simulink model "test_vacc_pkt_10_1"  (Simulink 7.2)
settings: Solver=ode45  StartTime=0.0  StopTime=90000  RelTol=1e-3
libraries: xbsIndex_r4 x802, xps_library x17, casper_library_misc x10, xbsReplacements_r4 x9
(part 2 of 6)

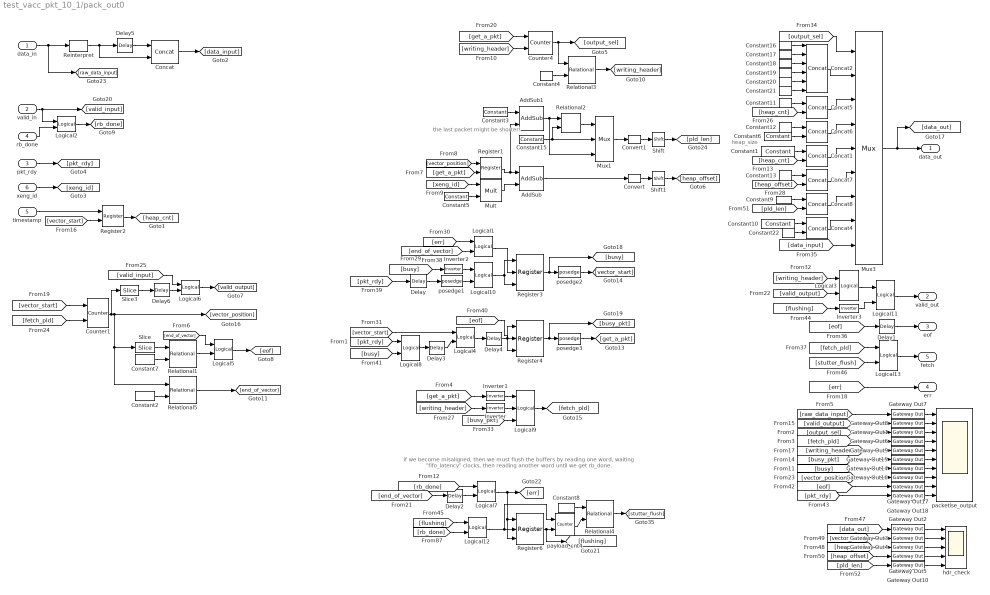
== system test_vacc_pkt_10_1/pack_out0 ==
  note: heap_size
  note: if we become misaligned,
      | then we must flush the buffers
      | by reading one word, waiting "fifo_latency" clocks,
      | then reading another word until we get rb_done.
  note: the last packet
      | might be shorter!
  data_in : Inport  OutDataType=sfix(16)  OutScaling=2^0
  valid_in : Inport  Port=2  OutDataType=sfix(16)  OutScaling=2^0
  pkt_rdy : Inport  Port=3  OutDataType=sfix(16)  OutScaling=2^0
  rb_done : Inport  Port=4  OutDataType=sfix(16)  OutScaling=2^0
  timestamp : Inport  Port=5  OutDataType=sfix(16)  OutScaling=2^0
  xeng_id : Inport  Port=6  OutDataType=sfix(16)  OutScaling=2^0
  AddSub : xbsIndex_r4/AddSub  mode=Addition  use_carryin=off  use_carryout=off  en=off  latency=1  precision=Full  arith_type=Unsigned  n_bits=16  bin_pt=14  quantization=Truncate  overflow=Wrap  dbl_ovrd=off  use_behavioral_HDL=on  hw_selection=Fabric  pipelined=off  block_type=addsub
  AddSub1 : xbsIndex_r4/AddSub  mode=Subtraction  use_carryin=off  use_carryout=off  en=off  latency=1  precision=Full  arith_type=Unsigned  n_bits=pkt_bits+4  bin_pt=0  quantization=Truncate  overflow=Wrap  dbl_ovrd=off  use_behavioral_HDL=on  hw_selection=Fabric  pipelined=off  block_type=addsub
  Concat{,1,4..8} (7 alike) : xbsIndex_r4/Concat  num_inputs=2  dbl_ovrd=off  block_type=concat
      settings: block_version=10.1.3
  Concat2 : xbsIndex_r4/Concat  num_inputs=6  dbl_ovrd=off  block_type=concat
      settings: block_version=10.1.3
  Constant1 : xbsIndex_r4/Constant  arith_type=Unsigned  const=5632 + 2^(spead_msw-spead_lsw-1)  n_bits=spead_msw-spead_lsw  bin_pt=0  explicit_period=on  period=1  equ=P=C  opselect=C  inp2=PCIN>>17  opr=+  inp1=P  carry=CIN  dbl_ovrd=off  block_type=constant
  Constant10 : xbsIndex_r4/Constant  arith_type=Unsigned  const=spead_item  n_bits=spead_msw-spead_lsw  bin_pt=0  explicit_period=on  period=1  equ=P=C  opselect=C  inp2=PCIN>>17  opr=+  inp1=P  carry=CIN  dbl_ovrd=off  block_type=constant
  Constant11 : xbsIndex_r4/Constant  arith_type=Unsigned  const=1 + 2^(spead_msw-spead_lsw-1)  n_bits=spead_msw-spead_lsw  bin_pt=0  explicit_period=on  period=1  equ=P=C  opselect=C  inp2=PCIN>>17  opr=+  inp1=P  carry=CIN  dbl_ovrd=off  block_type=constant
  Constant12 : xbsIndex_r4/Constant  arith_type=Unsigned  const="2 +  + 2^(spead_msw-spead_lsw-1)"  n_bits=spead_msw-spead_lsw  bin_pt=0  explicit_period=on  period=1  equ=P=C  opselect=C  inp2=PCIN>>17  opr=+  inp1=P  carry=CIN  dbl_ovrd=off  block_type=constant
  Constant13 : xbsIndex_r4/Constant  arith_type=Unsigned  const=3 + 2^(spead_msw-spead_lsw-1)  n_bits=spead_msw-spead_lsw  bin_pt=0  explicit_period=on  period=1  equ=P=C  opselect=C  inp2=PCIN>>17  opr=+  inp1=P  carry=CIN  dbl_ovrd=off  block_type=constant
  Constant15 : xbsIndex_r4/Constant  arith_type=Unsigned  const=(pkt_len*2)  n_bits=pkt_bits+2  bin_pt=0  explicit_period=on  period=1  equ=P=C  opselect=C  inp2=PCIN>>17  opr=+  inp1=P  carry=CIN  dbl_ovrd=off  block_type=constant
  Constant16 : xbsIndex_r4/Constant  arith_type=Unsigned  const=83  n_bits=8  bin_pt=0  explicit_period=on  period=1  equ=P=C  opselect=C  inp2=PCIN>>17  opr=+  inp1=P  carry=CIN  dbl_ovrd=off  block_type=constant
  Constant17 : xbsIndex_r4/Constant  arith_type=Unsigned  const=4  n_bits=8  bin_pt=0  explicit_period=on  period=1  equ=P=C  opselect=C  inp2=PCIN>>17  opr=+  inp1=P  carry=CIN  dbl_ovrd=off  block_type=constant
  Constant18 : xbsIndex_r4/Constant  arith_type=Unsigned  const=(spead_msw-spead_lsw)/8  n_bits=8  bin_pt=0  explicit_period=on  period=1  equ=P=C  opselect=C  inp2=PCIN>>17  opr=+  inp1=P  carry=CIN  dbl_ovrd=off  block_type=constant
  Constant19 : xbsIndex_r4/Constant  arith_type=Unsigned  const=spead_lsw/8  n_bits=8  bin_pt=0  explicit_period=on  period=1  equ=P=C  opselect=C  inp2=PCIN>>17  opr=+  inp1=P  carry=CIN  dbl_ovrd=off  block_type=constant
  Constant2 : xbsIndex_r4/Constant  arith_type=Unsigned  const=(vector_len)-1  n_bits=vector_bits+1  bin_pt=0  explicit_period=on  period=1  equ=P=C  opselect=C  inp2=PCIN>>17  opr=+  inp1=P  carry=CIN  dbl_ovrd=off  block_type=constant
  Constant20 : xbsIndex_r4/Constant  arith_type=Unsigned  const=0  n_bits=16  bin_pt=0  explicit_period=on  period=1  equ=P=C  opselect=C  inp2=PCIN>>17  opr=+  inp1=P  carry=CIN  dbl_ovrd=off  block_type=constant
  Constant21 : xbsIndex_r4/Constant  arith_type=Unsigned  const=6  n_bits=16  bin_pt=0  explicit_period=on  period=1  equ=P=C  opselect=C  inp2=PCIN>>17  opr=+  inp1=P  carry=CIN  dbl_ovrd=off  block_type=constant
  Constant22 : xbsIndex_r4/Constant  arith_type=Unsigned  const=0  n_bits=spead_lsw  bin_pt=0  explicit_period=on  period=1  equ=P=C  opselect=C  inp2=PCIN>>17  opr=+  inp1=P  carry=CIN  dbl_ovrd=off  block_type=constant
  Constant3 : xbsIndex_r4/Constant  arith_type=Unsigned  const=vector_len  n_bits=vector_bits+1  bin_pt=0  explicit_period=on  period=1  equ=P=C  opselect=C  inp2=PCIN>>17  opr=+  inp1=P  carry=CIN  dbl_ovrd=off  block_type=constant
  Constant4 : xbsIndex_r4/Constant  arith_type=Unsigned  const=7  n_bits=3  bin_pt=0  explicit_period=on  period=1  equ=P=C  opselect=C  inp2=PCIN>>17  opr=+  inp1=P  carry=CIN  dbl_ovrd=off  block_type=constant
  Constant5 : xbsIndex_r4/Constant  arith_type=Unsigned  const=vector_len  n_bits=vector_bits+1  bin_pt=0  explicit_period=on  period=1  equ=P=C  opselect=C  inp2=PCIN>>17  opr=+  inp1=P  carry=CIN  dbl_ovrd=off  block_type=constant
  Constant6 : xbsIndex_r4/Constant  arith_type=Unsigned  const=heap_len  n_bits=spead_lsw  bin_pt=0  explicit_period=on  period=1  equ=P=C  opselect=C  inp2=PCIN>>17  opr=+  inp1=P  carry=CIN  dbl_ovrd=off  block_type=constant
  Constant7 : xbsIndex_r4/Constant  arith_type=Unsigned  const=(pkt_len*2)-1  n_bits=pkt_bits+1  bin_pt=0  explicit_period=on  period=1  equ=P=C  opselect=C  inp2=PCIN>>17  opr=+  inp1=P  carry=CIN  dbl_ovrd=off  block_type=constant
  Constant8 : xbsIndex_r4/Constant  arith_type=Unsigned  const=1  n_bits=ceil(log2(fifo_latency))+1  bin_pt=0  explicit_period=on  period=1  equ=P=C  opselect=C  inp2=PCIN>>17  opr=+  inp1=P  carry=CIN  dbl_ovrd=off  block_type=constant
  Constant9 : xbsIndex_r4/Constant  arith_type=Unsigned  const=4 + 2^(spead_msw-spead_lsw-1)  n_bits=spead_msw-spead_lsw  bin_pt=0  explicit_period=on  period=1  equ=P=C  opselect=C  inp2=PCIN>>17  opr=+  inp1=P  carry=CIN  dbl_ovrd=off  block_type=constant
  Convert : xbsIndex_r4/Convert  arith_type=Unsigned  n_bits=spead_lsw  bin_pt=0  quantization=Truncate  overflow=Wrap  latency=0  dbl_ovrd=off  pipeline=off  block_type=convert
      settings: block_version=11.4
  Convert1 : xbsIndex_r4/Convert  arith_type=Unsigned  n_bits=spead_lsw  bin_pt=0  quantization=Truncate  overflow=Wrap  latency=0  dbl_ovrd=off  pipeline=off  block_type=convert
      settings: block_version=11.4
  Counter1 : xbsIndex_r4/Counter  cnt_type=Free Running  cnt_to=1023  operation=Up  start_count=0  cnt_by_val=1  arith_type=Unsigned  n_bits=vector_bits+1  bin_pt=0  load_pin=off  rst=on  en=on  explicit_period=on  period=1  dbl_ovrd=off  use_behavioral_HDL=off  implementation=Fabric  use_rpm=on  block_type=counter
      settings: xl_area=[0, 0, 0, 0, 0, 0, 0]
  Counter4 : xbsIndex_r4/Counter  cnt_type=Free Running  cnt_to=1023  operation=Up  start_count=0  cnt_by_val=1  arith_type=Unsigned  n_bits=3  bin_pt=0  load_pin=off  rst=on  en=on  explicit_period=on  period=1  dbl_ovrd=off  use_behavioral_HDL=off  implementation=Fabric  use_rpm=on  block_type=counter
      settings: xl_area=[0, 0, 0, 0, 0, 0, 0]
  Delay : xbsIndex_r4/Delay  en=off  latency=1  dbl_ovrd=off  reg_retiming=on  block_type=delay
      settings: block_version=11.4
  Delay{1..2,4,6} (4 alike) : xbsIndex_r4/Delay  en=off  latency=fifo_latency  dbl_ovrd=off  reg_retiming=on  block_type=delay
      settings: block_version=11.4
  Delay3 : xbsIndex_r4/Delay  en=off  latency=1  dbl_ovrd=off  reg_retiming=on  block_type=delay
      settings: block_version=11.4
  Delay5 : xbsIndex_r4/Delay  en=off  latency=1  dbl_ovrd=off  reg_retiming=on  block_type=delay
      settings: block_version=11.4
  Gateway Out{1..10,14..18} (15 alike) : xbsIndex_r4/Gateway Out  hdl_port=on  timing_constraint=None  locs_specified=off  LOCs={}  block_type=gatewayout
      settings: infoedit="Gateway out block.  Converts Xilinx fixed point inputs into ouputs of type Simulink integer, double, or fixed point.<P><P>Hardware notes:  In hardware these blocks become top level output ports or are discarded, depending on how they are configured."  xl_area=[0, 0, 0, 0, 0, 0, 0]  block_version=10.1.3
  Inverter{,1..3} (4 alike) : xbsIndex_r4/Inverter  en=off  latency=0  dbl_ovrd=off  block_type=inv
      settings: block_version=11.4
  Logical{1,3..5,13} (5 alike) : xbsIndex_r4/Logical  logical_function=OR  inputs=2  en=off  latency=0  precision=Full  arith_type=Unsigned  n_bits=8  bin_pt=2  align_bp=on  dbl_ovrd=off  block_type=logical
      settings: xl_area=[0, 0, 0, 0, 0, 0, 0]
  Logical{2,6,8,10..12} (6 alike) : xbsIndex_r4/Logical  logical_function=AND  inputs=2  en=off  latency=0  precision=Full  arith_type=Unsigned  n_bits=8  bin_pt=2  align_bp=on  dbl_ovrd=off  block_type=logical
      settings: xl_area=[0, 0, 0, 0, 0, 0, 0]
  Logical7 : xbsIndex_r4/Logical  logical_function=XOR  inputs=2  en=off  latency=0  precision=Full  arith_type=Unsigned  n_bits=8  bin_pt=2  align_bp=on  dbl_ovrd=off  block_type=logical
      settings: xl_area=[0, 0, 0, 0, 0, 0, 0]
  Logical9 : xbsIndex_r4/Logical  logical_function=AND  inputs=3  en=off  latency=0  precision=Full  arith_type=Unsigned  n_bits=8  bin_pt=2  align_bp=on  dbl_ovrd=off  block_type=logical
      settings: xl_area=[0, 0, 0, 0, 0, 0, 0]
  Mult : xbsIndex_r4/Mult  precision=Full  arith_type="Signed  (2's comp)"  n_bits=16  bin_pt=14  quantization=Truncate  overflow=Wrap  en=off  latency=3  dbl_ovrd=off  use_behavioral_HDL=on  opt=Speed  use_embedded=on  optimum_pipeline=on  pipeline=on  use_rpm=on  placement_style=Triangular  block_type=mult
      settings: block_version=11.4
  Mux1 : xbsIndex_r4/Mux  inputs=2  en=off  latency=1  precision=Full  arith_type="Signed  (2's comp)"  n_bits=8  bin_pt=2  quantization=Truncate  overflow=Wrap  dbl_ovrd=off  block_type=mux
      settings: xl_area=[0, 0, 0, 0, 0, 0, 0]
  Mux3 : xbsIndex_r4/Mux  inputs=8  en=off  latency=0  precision=Full  arith_type="Signed  (2's comp)"  n_bits=8  bin_pt=2  quantization=Truncate  overflow=Wrap  dbl_ovrd=off  block_type=mux
      settings: xl_area=[0, 0, 0, 0, 0, 0, 0]
  Register1 : xbsIndex_r4/Register  init=0  rst=off  en=on  dbl_ovrd=off  block_type=register
  Register2 : xbsIndex_r4/Register  init=0  rst=off  en=on  dbl_ovrd=off  block_type=register
  Register3 : xbsIndex_r4/Register  init=0  rst=on  en=on  dbl_ovrd=off  block_type=register
  Register4 : xbsIndex_r4/Register  init=0  rst=on  en=on  dbl_ovrd=off  block_type=register
  Register6 : xbsIndex_r4/Register  init=0  rst=on  en=on  dbl_ovrd=off  block_type=register
      settings: xl_area=[0, 0, 0, 0, 0, 0, 0]
  Reinterpret : xbsIndex_r4/Reinterpret  force_arith_type=on  arith_type=Unsigned  force_bin_pt=on  bin_pt=0  block_type=reinterpret
      settings: infoedit="Changes signal type without altering the binary representation.   You can changed the signal between signed and unsigned, and relocate the binary point.<br><br>Hardware notes: In hardware this block costs nothing.<br><br>Example:  Suppose the input is 6 bits wide, signed, with 2 fractional bits, and the output is forced to unsigned with 0 fractional bits.  Then an input of -2.0 (1110.00 in binary 2's complement) becomes an output of 56 (111000 in binary)."
  Relational1 : xbsIndex_r4/Relational  mode=a=b  en=off  latency=0  dbl_ovrd=off  block_type=relational
      settings: xl_area=[0, 0, 0, 0, 0, 0, 0]  block_version=10.1.3
  Relational2 : xbsIndex_r4/Relational  mode=a<b  en=off  latency=0  dbl_ovrd=off  block_type=relational
      settings: xl_area=[0, 0, 0, 0, 0, 0, 0]  block_version=10.1.3
  Relational3 : xbsIndex_r4/Relational  mode=a<b  en=off  latency=0  dbl_ovrd=off  block_type=relational
      settings: xl_area=[0, 0, 0, 0, 0, 0, 0]  block_version=10.1.3
  Relational4 : xbsIndex_r4/Relational  mode=a=b  en=off  latency=0  dbl_ovrd=off  block_type=relational
      settings: xl_area=[0, 0, 0, 0, 0, 0, 0]  block_version=10.1.3
  Relational5 : xbsIndex_r4/Relational  mode=a=b  en=off  latency=0  dbl_ovrd=off  block_type=relational
      settings: xl_area=[0, 0, 0, 0, 0, 0, 0]  block_version=10.1.3
  Shift : xbsIndex_r4/Shift  shift_dir=Left  shift_bits=2  en=off  latency=0  precision=Full  arith_type="Signed  (2's comp)"  n_bits=16  bin_pt=14  quantization=Truncate  overflow=Wrap  dbl_ovrd=off  block_type=shift
  Shift1 : xbsIndex_r4/Shift  shift_dir=Left  shift_bits=2  en=off  latency=0  precision=Full  arith_type="Signed  (2's comp)"  n_bits=16  bin_pt=14  quantization=Truncate  overflow=Wrap  dbl_ovrd=off  block_type=shift
  Slice : xbsIndex_r4/Slice  nbits=pkt_bits+1  boolean_output=off  mode=Lower Bit Location + Width  bit1=0  base1=MSB of Input  bit0=0  base0=LSB of Input  dbl_ovrd=off  block_type=slice
  Slice3 : xbsIndex_r4/Slice  nbits=1  boolean_output=on  mode=Lower Bit Location + Width  bit1=0  base1=MSB of Input  bit0=0  base0=LSB of Input  dbl_ovrd=off  block_type=slice
  hdr_check : Scope  NumInputPorts=5
      settings: YMin=0~0~0~0~920  YMax=1e+19~1~17500~3250~1030  SaveName=ScopeData12
  packetise_output : Scope  NumInputPorts=10
      settings: YMin=1000~-1~7~-1~-1~-1~-1~1024~-1~-1  YMax=1000~1~7~1~1~1~1~1024~1~1
  payload_cnt4 : xbsIndex_r4/Counter  cnt_type=Count Limited  cnt_to=max((fifo_latency + 1),2)  operation=Up  start_count=0  cnt_by_val=1  arith_type=Unsigned  n_bits=ceil(log2(fifo_latency))+1  bin_pt=0  load_pin=off  rst=on  en=on  explicit_period=on  period=1  dbl_ovrd=off  use_behavioral_HDL=off  implementation=Fabric  use_rpm=on  block_type=counter
      settings: xl_area=[0, 0, 0, 0, 0, 0, 0]
  posedge1 : casper_library_misc/posedge  Tag=Rising Edge Detector  SystemSampleTime=-1
  posedge2 : casper_library_misc/posedge  Tag=Rising Edge Detector  SystemSampleTime=-1
  posedge3 : casper_library_misc/posedge  Tag=Rising Edge Detector  SystemSampleTime=-1
  data_out : Outport  OutDataType=sfix(16)  OutScaling=2^0
  valid_out : Outport  Port=2  OutDataType=sfix(16)  OutScaling=2^0
  eof : Outport  Port=3  OutDataType=sfix(16)  OutScaling=2^0
  err : Outport  Port=4  OutDataType=sfix(16)  OutScaling=2^0
  fetch : Outport  Port=5  OutDataType=sfix(16)  OutScaling=2^0
  wires:
  Gateway Out14/1 -> packetise_output/7
  [end_of_vector] -> Logical5/1
  Gateway Out15/1 -> packetise_output/6
  Gateway Out9/1 -> packetise_output/5
  Gateway Out6/1 -> packetise_output/4
  Gateway Out1/1 -> packetise_output/3
  Gateway Out8/1 -> packetise_output/2
  Gateway Out7/1 -> packetise_output/1
  Logical5/1 -> [eof]
  Logical2/1 -> [rb_done]
  xeng_id/1 -> [xeng_id]
  Concat/1 -> [data_input]
  Gateway Out16/1 -> packetise_output/8
  Slice/1 -> Relational1/1
  Counter1/1 -> Slice3/1, [vector_position], Slice/1, Relational5/1
  timestamp/1 -> Register2/1
  Register2/1 -> [heap_cnt]
  [vector_start] -> Register2/2
  Constant2/1 -> Relational5/2
  Relational5/1 -> [end_of_vector]
  data_in/1 -> Reinterpret/1, [raw_data_input]
  valid_in/1 -> Logical2/1, [valid_input]
  pkt_rdy/1 -> [pkt_rdy]
  Reinterpret/1 -> Delay5/1, Concat/2
  rb_done/1 -> Logical2/2
  Delay5/1 -> Concat/1
  Gateway Out17/1 -> packetise_output/9
  Gateway Out18/1 -> packetise_output/10
  Slice3/1 -> Delay6/1
  Delay6/1 -> Logical6/2
  Logical6/1 -> [valid_output]
  [valid_input] -> Logical6/1
  [fetch_pld] -> Counter1/2
  [vector_start] -> Counter1/1
  Constant7/1 -> Relational1/2
  Relational1/1 -> Logical5/2
  [fetch_pld] -> Gateway Out6/1
  [writing_header] -> Gateway Out9/1
  [busy] -> Gateway Out14/1
  [valid_output] -> Gateway Out8/1
  [busy_pkt] -> Gateway Out15/1
  [output_sel] -> Gateway Out1/1
  [raw_data_input] -> Gateway Out7/1
  [vector_position] -> Gateway Out16/1
  Mux3/1 -> [data_out], data_out/1
  [output_sel] -> Mux3/1
  Concat2/1 -> Mux3/2
  Constant16/1 -> Concat2/1
  Constant17/1 -> Concat2/2
  Constant18/1 -> Concat2/3
  Constant19/1 -> Concat2/4
  [data_input] -> Mux3/9
  [writing_header] -> Logical3/1
  [eof] -> Delay1/1
  Delay1/1 -> eof/1
  Constant20/1 -> Concat2/5
  Constant21/1 -> Concat2/6
  Concat4/1 -> Mux3/8
  Constant22/1 -> Concat4/2
  Constant10/1 -> Concat4/1
  Constant11/1 -> Concat5/1
  [heap_cnt] -> Concat5/2
  Concat5/1 -> Mux3/3
  Constant12/1 -> Concat6/1
  Constant6/1 -> Concat6/2
  Concat6/1 -> Mux3/4
  Constant13/1 -> Concat7/1
  [heap_offset] -> Concat7/2
  Concat1/1 -> Mux3/5
  Concat7/1 -> Mux3/6
  [pld_len] -> Concat8/2
  Constant9/1 -> Concat8/1
  [valid_output] -> Logical3/2
  Counter4/1 -> Relational3/1, [output_sel]
  Relational3/1 -> [writing_header]
  Constant4/1 -> Relational3/2
  [writing_header] -> Counter4/2
  [vector_position] -> Register1/1
  Register1/1 -> AddSub1/2, AddSub/1
  [heap_cnt] -> Concat1/2
  Constant1/1 -> Concat1/1
  [get_a_pkt] -> Register1/2
  [err] -> err/1
  [rb_done] -> Logical7/1
  [end_of_vector] -> Delay2/1
  Constant5/1 -> Mult/2
  [xeng_id] -> Mult/1
  Mult/1 -> AddSub/2
  AddSub/1 -> Convert/1
  Convert/1 -> Shift1/1
  [get_a_pkt] -> Counter4/1
  [writing_header] -> Inverter/1
  [vector_start] -> Logical4/1
  Logical4/1 -> Delay4/1
  [pkt_rdy] -> Logical8/1
  Logical8/1 -> Delay3/1
  Register3/1 -> [busy], posedge2/1
  posedge2/1 -> [vector_start]
  Inverter2/1 -> Logical10/1
  Logical10/1 -> Register3/1, Register3/3
  [end_of_vector] -> Logical1/2
  [pkt_rdy] -> Delay/1
  posedge1/1 -> Logical10/2
  [busy] -> Inverter2/1
  Delay/1 -> posedge1/1
  Delay2/1 -> Logical7/2
  [get_a_pkt] -> Inverter1/1
  Delay3/1 -> Logical4/2
  Delay4/1 -> Register4/3, Register4/1
  posedge3/1 -> [get_a_pkt]
  Register4/1 -> posedge3/1, [busy_pkt]
  [eof] -> Register4/2
  [busy] -> Logical8/2
  Inverter1/1 -> Logical9/1
  Inverter/1 -> Logical9/2
  [busy_pkt] -> Logical9/3
  Logical9/1 -> [fetch_pld]
  [eof] -> Gateway Out17/1
  [pkt_rdy] -> Gateway Out18/1
  Logical7/1 -> Register6/3, Register6/1, [err]
  [rb_done] -> Logical12/2
  payload_cnt4/1 -> Relational4/2
  Constant8/1 -> Relational4/1
  Register6/1 -> payload_cnt4/2, [flushing]
  Relational4/1 -> [stutter_flush]
  Logical1/1 -> Register3/2
  [err] -> Logical1/1
  Logical3/1 -> Logical11/1
  Logical11/1 -> valid_out/1
  Inverter3/1 -> Logical11/2
  [flushing] -> Inverter3/1
  Logical12/1 -> payload_cnt4/1, Register6/2
  [flushing] -> Logical12/1
  Logical13/1 -> fetch/1
  [fetch_pld] -> Logical13/1
  [stutter_flush] -> Logical13/2
  [data_out] -> Gateway Out2/1
  [vector_start] -> Gateway Out3/1
  [heap_cnt] -> Gateway Out4/1
  [heap_offset] -> Gateway Out5/1
  Gateway Out2/1 -> hdr_check/1
  Gateway Out3/1 -> hdr_check/2
  Gateway Out4/1 -> hdr_check/3
  Gateway Out5/1 -> hdr_check/4
  Constant15/1 -> Mux1/2, Relational2/2
  Concat8/1 -> Mux3/7
  Mux1/1 -> Convert1/1
  Relational2/1 -> Mux1/1
  Constant3/1 -> AddSub1/1
  AddSub1/1 -> Relational2/1, Mux1/3
  Convert1/1 -> Shift/1
  Shift/1 -> [pld_len]
  Shift1/1 -> [heap_offset]
  Gateway Out10/1 -> hdr_check/5
  [pld_len] -> Gateway Out10/1

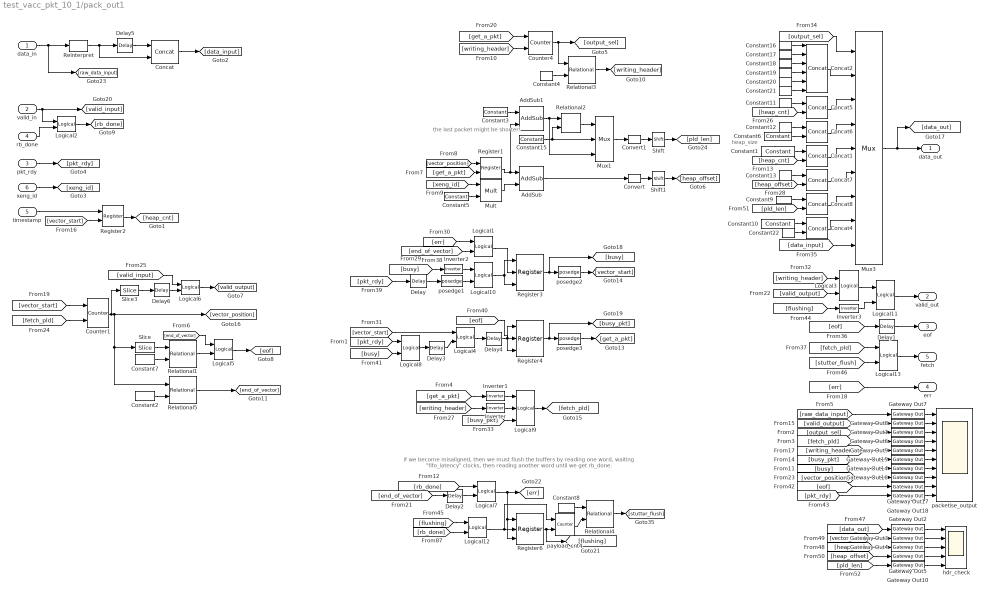
== system test_vacc_pkt_10_1/pack_out1 ==
  note: the last packet
      | might be shorter!
  note: if we become misaligned,
      | then we must flush the buffers
      | by reading one word, waiting "fifo_latency" clocks,
      | then reading another word until we get rb_done.
  note: heap_size
  data_in : Inport  OutDataType=sfix(16)  OutScaling=2^0
  valid_in : Inport  Port=2  OutDataType=sfix(16)  OutScaling=2^0
  pkt_rdy : Inport  Port=3  OutDataType=sfix(16)  OutScaling=2^0
  rb_done : Inport  Port=4  OutDataType=sfix(16)  OutScaling=2^0
  timestamp : Inport  Port=5  OutDataType=sfix(16)  OutScaling=2^0
  xeng_id : Inport  Port=6  OutDataType=sfix(16)  OutScaling=2^0
  AddSub : xbsIndex_r4/AddSub  mode=Addition  use_carryin=off  use_carryout=off  en=off  latency=1  precision=Full  arith_type=Unsigned  n_bits=16  bin_pt=14  quantization=Truncate  overflow=Wrap  dbl_ovrd=off  use_behavioral_HDL=on  hw_selection=Fabric  pipelined=off  block_type=addsub
  AddSub1 : xbsIndex_r4/AddSub  mode=Subtraction  use_carryin=off  use_carryout=off  en=off  latency=1  precision=Full  arith_type=Unsigned  n_bits=pkt_bits+4  bin_pt=0  quantization=Truncate  overflow=Wrap  dbl_ovrd=off  use_behavioral_HDL=on  hw_selection=Fabric  pipelined=off  block_type=addsub
  Concat{,1,4..8} (7 alike) : xbsIndex_r4/Concat  num_inputs=2  dbl_ovrd=off  block_type=concat
      settings: block_version=10.1.3
  Concat2 : xbsIndex_r4/Concat  num_inputs=6  dbl_ovrd=off  block_type=concat
      settings: block_version=10.1.3
  Constant1 : xbsIndex_r4/Constant  arith_type=Unsigned  const=5632 + 2^(spead_msw-spead_lsw-1)  n_bits=spead_msw-spead_lsw  bin_pt=0  explicit_period=on  period=1  equ=P=C  opselect=C  inp2=PCIN>>17  opr=+  inp1=P  carry=CIN  dbl_ovrd=off  block_type=constant
  Constant10 : xbsIndex_r4/Constant  arith_type=Unsigned  const=spead_item  n_bits=spead_msw-spead_lsw  bin_pt=0  explicit_period=on  period=1  equ=P=C  opselect=C  inp2=PCIN>>17  opr=+  inp1=P  carry=CIN  dbl_ovrd=off  block_type=constant
  Constant11 : xbsIndex_r4/Constant  arith_type=Unsigned  const=1 + 2^(spead_msw-spead_lsw-1)  n_bits=spead_msw-spead_lsw  bin_pt=0  explicit_period=on  period=1  equ=P=C  opselect=C  inp2=PCIN>>17  opr=+  inp1=P  carry=CIN  dbl_ovrd=off  block_type=constant
  Constant12 : xbsIndex_r4/Constant  arith_type=Unsigned  const="2 +  + 2^(spead_msw-spead_lsw-1)"  n_bits=spead_msw-spead_lsw  bin_pt=0  explicit_period=on  period=1  equ=P=C  opselect=C  inp2=PCIN>>17  opr=+  inp1=P  carry=CIN  dbl_ovrd=off  block_type=constant
  Constant13 : xbsIndex_r4/Constant  arith_type=Unsigned  const=3 + 2^(spead_msw-spead_lsw-1)  n_bits=spead_msw-spead_lsw  bin_pt=0  explicit_period=on  period=1  equ=P=C  opselect=C  inp2=PCIN>>17  opr=+  inp1=P  carry=CIN  dbl_ovrd=off  block_type=constant
  Constant15 : xbsIndex_r4/Constant  arith_type=Unsigned  const=(pkt_len*2)  n_bits=pkt_bits+2  bin_pt=0  explicit_period=on  period=1  equ=P=C  opselect=C  inp2=PCIN>>17  opr=+  inp1=P  carry=CIN  dbl_ovrd=off  block_type=constant
  Constant16 : xbsIndex_r4/Constant  arith_type=Unsigned  const=83  n_bits=8  bin_pt=0  explicit_period=on  period=1  equ=P=C  opselect=C  inp2=PCIN>>17  opr=+  inp1=P  carry=CIN  dbl_ovrd=off  block_type=constant
  Constant17 : xbsIndex_r4/Constant  arith_type=Unsigned  const=4  n_bits=8  bin_pt=0  explicit_period=on  period=1  equ=P=C  opselect=C  inp2=PCIN>>17  opr=+  inp1=P  carry=CIN  dbl_ovrd=off  block_type=constant
  Constant18 : xbsIndex_r4/Constant  arith_type=Unsigned  const=(spead_msw-spead_lsw)/8  n_bits=8  bin_pt=0  explicit_period=on  period=1  equ=P=C  opselect=C  inp2=PCIN>>17  opr=+  inp1=P  carry=CIN  dbl_ovrd=off  block_type=constant
  Constant19 : xbsIndex_r4/Constant  arith_type=Unsigned  const=spead_lsw/8  n_bits=8  bin_pt=0  explicit_period=on  period=1  equ=P=C  opselect=C  inp2=PCIN>>17  opr=+  inp1=P  carry=CIN  dbl_ovrd=off  block_type=constant
  Constant2 : xbsIndex_r4/Constant  arith_type=Unsigned  const=(vector_len)-1  n_bits=vector_bits+1  bin_pt=0  explicit_period=on  period=1  equ=P=C  opselect=C  inp2=PCIN>>17  opr=+  inp1=P  carry=CIN  dbl_ovrd=off  block_type=constant
  Constant20 : xbsIndex_r4/Constant  arith_type=Unsigned  const=0  n_bits=16  bin_pt=0  explicit_period=on  period=1  equ=P=C  opselect=C  inp2=PCIN>>17  opr=+  inp1=P  carry=CIN  dbl_ovrd=off  block_type=constant
  Constant21 : xbsIndex_r4/Constant  arith_type=Unsigned  const=6  n_bits=16  bin_pt=0  explicit_period=on  period=1  equ=P=C  opselect=C  inp2=PCIN>>17  opr=+  inp1=P  carry=CIN  dbl_ovrd=off  block_type=constant
  Constant22 : xbsIndex_r4/Constant  arith_type=Unsigned  const=0  n_bits=spead_lsw  bin_pt=0  explicit_period=on  period=1  equ=P=C  opselect=C  inp2=PCIN>>17  opr=+  inp1=P  carry=CIN  dbl_ovrd=off  block_type=constant
  Constant3 : xbsIndex_r4/Constant  arith_type=Unsigned  const=vector_len  n_bits=vector_bits+1  bin_pt=0  explicit_period=on  period=1  equ=P=C  opselect=C  inp2=PCIN>>17  opr=+  inp1=P  carry=CIN  dbl_ovrd=off  block_type=constant
  Constant4 : xbsIndex_r4/Constant  arith_type=Unsigned  const=7  n_bits=3  bin_pt=0  explicit_period=on  period=1  equ=P=C  opselect=C  inp2=PCIN>>17  opr=+  inp1=P  carry=CIN  dbl_ovrd=off  block_type=constant
  Constant5 : xbsIndex_r4/Constant  arith_type=Unsigned  const=vector_len  n_bits=vector_bits+1  bin_pt=0  explicit_period=on  period=1  equ=P=C  opselect=C  inp2=PCIN>>17  opr=+  inp1=P  carry=CIN  dbl_ovrd=off  block_type=constant
  Constant6 : xbsIndex_r4/Constant  arith_type=Unsigned  const=heap_len  n_bits=spead_lsw  bin_pt=0  explicit_period=on  period=1  equ=P=C  opselect=C  inp2=PCIN>>17  opr=+  inp1=P  carry=CIN  dbl_ovrd=off  block_type=constant
  Constant7 : xbsIndex_r4/Constant  arith_type=Unsigned  const=(pkt_len*2)-1  n_bits=pkt_bits+1  bin_pt=0  explicit_period=on  period=1  equ=P=C  opselect=C  inp2=PCIN>>17  opr=+  inp1=P  carry=CIN  dbl_ovrd=off  block_type=constant
  Constant8 : xbsIndex_r4/Constant  arith_type=Unsigned  const=1  n_bits=ceil(log2(fifo_latency))+1  bin_pt=0  explicit_period=on  period=1  equ=P=C  opselect=C  inp2=PCIN>>17  opr=+  inp1=P  carry=CIN  dbl_ovrd=off  block_type=constant
  Constant9 : xbsIndex_r4/Constant  arith_type=Unsigned  const=4 + 2^(spead_msw-spead_lsw-1)  n_bits=spead_msw-spead_lsw  bin_pt=0  explicit_period=on  period=1  equ=P=C  opselect=C  inp2=PCIN>>17  opr=+  inp1=P  carry=CIN  dbl_ovrd=off  block_type=constant
  Convert : xbsIndex_r4/Convert  arith_type=Unsigned  n_bits=spead_lsw  bin_pt=0  quantization=Truncate  overflow=Wrap  latency=0  dbl_ovrd=off  pipeline=off  block_type=convert
      settings: block_version=11.4
  Convert1 : xbsIndex_r4/Convert  arith_type=Unsigned  n_bits=spead_lsw  bin_pt=0  quantization=Truncate  overflow=Wrap  latency=0  dbl_ovrd=off  pipeline=off  block_type=convert
      settings: block_version=11.4
  Counter1 : xbsIndex_r4/Counter  cnt_type=Free Running  cnt_to=1023  operation=Up  start_count=0  cnt_by_val=1  arith_type=Unsigned  n_bits=vector_bits+1  bin_pt=0  load_pin=off  rst=on  en=on  explicit_period=on  period=1  dbl_ovrd=off  use_behavioral_HDL=off  implementation=Fabric  use_rpm=on  block_type=counter
      settings: xl_area=[0, 0, 0, 0, 0, 0, 0]
  Counter4 : xbsIndex_r4/Counter  cnt_type=Free Running  cnt_to=1023  operation=Up  start_count=0  cnt_by_val=1  arith_type=Unsigned  n_bits=3  bin_pt=0  load_pin=off  rst=on  en=on  explicit_period=on  period=1  dbl_ovrd=off  use_behavioral_HDL=off  implementation=Fabric  use_rpm=on  block_type=counter
      settings: xl_area=[0, 0, 0, 0, 0, 0, 0]
  Delay : xbsIndex_r4/Delay  en=off  latency=1  dbl_ovrd=off  reg_retiming=on  block_type=delay
      settings: block_version=11.4
  Delay{1..2,4,6} (4 alike) : xbsIndex_r4/Delay  en=off  latency=fifo_latency  dbl_ovrd=off  reg_retiming=on  block_type=delay
      settings: block_version=11.4
  Delay3 : xbsIndex_r4/Delay  en=off  latency=1  dbl_ovrd=off  reg_retiming=on  block_type=delay
      settings: block_version=11.4
  Delay5 : xbsIndex_r4/Delay  en=off  latency=1  dbl_ovrd=off  reg_retiming=on  block_type=delay
      settings: block_version=11.4
  Gateway Out{1..10,14..18} (15 alike) : xbsIndex_r4/Gateway Out  hdl_port=on  timing_constraint=None  locs_specified=off  LOCs={}  block_type=gatewayout
      settings: infoedit="Gateway out block.  Converts Xilinx fixed point inputs into ouputs of type Simulink integer, double, or fixed point.<P><P>Hardware notes:  In hardware these blocks become top level output ports or are discarded, depending on how they are configured."  xl_area=[0, 0, 0, 0, 0, 0, 0]  block_version=10.1.3
  Inverter{,1..3} (4 alike) : xbsIndex_r4/Inverter  en=off  latency=0  dbl_ovrd=off  block_type=inv
      settings: block_version=11.4
  Logical{1,3..5,13} (5 alike) : xbsIndex_r4/Logical  logical_function=OR  inputs=2  en=off  latency=0  precision=Full  arith_type=Unsigned  n_bits=8  bin_pt=2  align_bp=on  dbl_ovrd=off  block_type=logical
      settings: xl_area=[0, 0, 0, 0, 0, 0, 0]
  Logical{2,6,8,10..12} (6 alike) : xbsIndex_r4/Logical  logical_function=AND  inputs=2  en=off  latency=0  precision=Full  arith_type=Unsigned  n_bits=8  bin_pt=2  align_bp=on  dbl_ovrd=off  block_type=logical
      settings: xl_area=[0, 0, 0, 0, 0, 0, 0]
  Logical7 : xbsIndex_r4/Logical  logical_function=XOR  inputs=2  en=off  latency=0  precision=Full  arith_type=Unsigned  n_bits=8  bin_pt=2  align_bp=on  dbl_ovrd=off  block_type=logical
      settings: xl_area=[0, 0, 0, 0, 0, 0, 0]
  Logical9 : xbsIndex_r4/Logical  logical_function=AND  inputs=3  en=off  latency=0  precision=Full  arith_type=Unsigned  n_bits=8  bin_pt=2  align_bp=on  dbl_ovrd=off  block_type=logical
      settings: xl_area=[0, 0, 0, 0, 0, 0, 0]
  Mult : xbsIndex_r4/Mult  precision=Full  arith_type="Signed  (2's comp)"  n_bits=16  bin_pt=14  quantization=Truncate  overflow=Wrap  en=off  latency=3  dbl_ovrd=off  use_behavioral_HDL=on  opt=Speed  use_embedded=on  optimum_pipeline=on  pipeline=on  use_rpm=on  placement_style=Triangular  block_type=mult
      settings: block_version=11.4
  Mux1 : xbsIndex_r4/Mux  inputs=2  en=off  latency=1  precision=Full  arith_type="Signed  (2's comp)"  n_bits=8  bin_pt=2  quantization=Truncate  overflow=Wrap  dbl_ovrd=off  block_type=mux
      settings: xl_area=[0, 0, 0, 0, 0, 0, 0]
  Mux3 : xbsIndex_r4/Mux  inputs=8  en=off  latency=0  precision=Full  arith_type="Signed  (2's comp)"  n_bits=8  bin_pt=2  quantization=Truncate  overflow=Wrap  dbl_ovrd=off  block_type=mux
      settings: xl_area=[0, 0, 0, 0, 0, 0, 0]
  Register1 : xbsIndex_r4/Register  init=0  rst=off  en=on  dbl_ovrd=off  block_type=register
  Register2 : xbsIndex_r4/Register  init=0  rst=off  en=on  dbl_ovrd=off  block_type=register
  Register3 : xbsIndex_r4/Register  init=0  rst=on  en=on  dbl_ovrd=off  block_type=register
  Register4 : xbsIndex_r4/Register  init=0  rst=on  en=on  dbl_ovrd=off  block_type=register
  Register6 : xbsIndex_r4/Register  init=0  rst=on  en=on  dbl_ovrd=off  block_type=register
      settings: xl_area=[0, 0, 0, 0, 0, 0, 0]
  Reinterpret : xbsIndex_r4/Reinterpret  force_arith_type=on  arith_type=Unsigned  force_bin_pt=on  bin_pt=0  block_type=reinterpret
      settings: infoedit="Changes signal type without altering the binary representation.   You can changed the signal between signed and unsigned, and relocate the binary point.<br><br>Hardware notes: In hardware this block costs nothing.<br><br>Example:  Suppose the input is 6 bits wide, signed, with 2 fractional bits, and the output is forced to unsigned with 0 fractional bits.  Then an input of -2.0 (1110.00 in binary 2's complement) becomes an output of 56 (111000 in binary)."
  Relational1 : xbsIndex_r4/Relational  mode=a=b  en=off  latency=0  dbl_ovrd=off  block_type=relational
      settings: xl_area=[0, 0, 0, 0, 0, 0, 0]  block_version=10.1.3
  Relational2 : xbsIndex_r4/Relational  mode=a<b  en=off  latency=0  dbl_ovrd=off  block_type=relational
      settings: xl_area=[0, 0, 0, 0, 0, 0, 0]  block_version=10.1.3
  Relational3 : xbsIndex_r4/Relational  mode=a<b  en=off  latency=0  dbl_ovrd=off  block_type=relational
      settings: xl_area=[0, 0, 0, 0, 0, 0, 0]  block_version=10.1.3
  Relational4 : xbsIndex_r4/Relational  mode=a=b  en=off  latency=0  dbl_ovrd=off  block_type=relational
      settings: xl_area=[0, 0, 0, 0, 0, 0, 0]  block_version=10.1.3
  Relational5 : xbsIndex_r4/Relational  mode=a=b  en=off  latency=0  dbl_ovrd=off  block_type=relational
      settings: xl_area=[0, 0, 0, 0, 0, 0, 0]  block_version=10.1.3
  Shift : xbsIndex_r4/Shift  shift_dir=Left  shift_bits=2  en=off  latency=0  precision=Full  arith_type="Signed  (2's comp)"  n_bits=16  bin_pt=14  quantization=Truncate  overflow=Wrap  dbl_ovrd=off  block_type=shift
  Shift1 : xbsIndex_r4/Shift  shift_dir=Left  shift_bits=2  en=off  latency=0  precision=Full  arith_type="Signed  (2's comp)"  n_bits=16  bin_pt=14  quantization=Truncate  overflow=Wrap  dbl_ovrd=off  block_type=shift
  Slice : xbsIndex_r4/Slice  nbits=pkt_bits+1  boolean_output=off  mode=Lower Bit Location + Width  bit1=0  base1=MSB of Input  bit0=0  base0=LSB of Input  dbl_ovrd=off  block_type=slice
  Slice3 : xbsIndex_r4/Slice  nbits=1  boolean_output=on  mode=Lower Bit Location + Width  bit1=0  base1=MSB of Input  bit0=0  base0=LSB of Input  dbl_ovrd=off  block_type=slice
  hdr_check : Scope  NumInputPorts=5
      settings: YMin=0~0~0~0~920  YMax=1e+19~1~17500~3250~1030  SaveName=ScopeData12
  packetise_output : Scope  NumInputPorts=10
      settings: YMin=1000~-1~7~-1~-1~-1~-1~1024~-1~-1  YMax=1000~1~7~1~1~1~1~1024~1~1
  payload_cnt4 : xbsIndex_r4/Counter  cnt_type=Count Limited  cnt_to=max((fifo_latency + 1),2)  operation=Up  start_count=0  cnt_by_val=1  arith_type=Unsigned  n_bits=ceil(log2(fifo_latency))+1  bin_pt=0  load_pin=off  rst=on  en=on  explicit_period=on  period=1  dbl_ovrd=off  use_behavioral_HDL=off  implementation=Fabric  use_rpm=on  block_type=counter
      settings: xl_area=[0, 0, 0, 0, 0, 0, 0]
  posedge1 : casper_library_misc/posedge  Tag=Rising Edge Detector  SystemSampleTime=-1
  posedge2 : casper_library_misc/posedge  Tag=Rising Edge Detector  SystemSampleTime=-1
  posedge3 : casper_library_misc/posedge  Tag=Rising Edge Detector  SystemSampleTime=-1
  data_out : Outport  OutDataType=sfix(16)  OutScaling=2^0
  valid_out : Outport  Port=2  OutDataType=sfix(16)  OutScaling=2^0
  eof : Outport  Port=3  OutDataType=sfix(16)  OutScaling=2^0
  err : Outport  Port=4  OutDataType=sfix(16)  OutScaling=2^0
  fetch : Outport  Port=5  OutDataType=sfix(16)  OutScaling=2^0
  wires:
  [pld_len] -> Gateway Out10/1
  Gateway Out10/1 -> hdr_check/5
  Shift1/1 -> [heap_offset]
  Shift/1 -> [pld_len]
  Convert1/1 -> Shift/1
  AddSub1/1 -> Mux1/3, Relational2/1
  Constant3/1 -> AddSub1/1
  Relational2/1 -> Mux1/1
  Mux1/1 -> Convert1/1
  Concat8/1 -> Mux3/7
  Constant15/1 -> Relational2/2, Mux1/2
  Gateway Out5/1 -> hdr_check/4
  Gateway Out4/1 -> hdr_check/3
  Gateway Out3/1 -> hdr_check/2
  Gateway Out2/1 -> hdr_check/1
  [heap_offset] -> Gateway Out5/1
  [heap_cnt] -> Gateway Out4/1
  [vector_start] -> Gateway Out3/1
  [data_out] -> Gateway Out2/1
  [stutter_flush] -> Logical13/2
  [fetch_pld] -> Logical13/1
  Logical13/1 -> fetch/1
  [flushing] -> Logical12/1
  Logical12/1 -> Register6/2, payload_cnt4/1
  [flushing] -> Inverter3/1
  Inverter3/1 -> Logical11/2
  Logical11/1 -> valid_out/1
  Logical3/1 -> Logical11/1
  [err] -> Logical1/1
  Logical1/1 -> Register3/2
  Relational4/1 -> [stutter_flush]
  Register6/1 -> [flushing], payload_cnt4/2
  Constant8/1 -> Relational4/1
  payload_cnt4/1 -> Relational4/2
  [rb_done] -> Logical12/2
  Logical7/1 -> [err], Register6/1, Register6/3
  [pkt_rdy] -> Gateway Out18/1
  [eof] -> Gateway Out17/1
  Logical9/1 -> [fetch_pld]
  [busy_pkt] -> Logical9/3
  Inverter/1 -> Logical9/2
  Inverter1/1 -> Logical9/1
  [busy] -> Logical8/2
  [eof] -> Register4/2
  Register4/1 -> [busy_pkt], posedge3/1
  posedge3/1 -> [get_a_pkt]
  Delay4/1 -> Register4/1, Register4/3
  Delay3/1 -> Logical4/2
  [get_a_pkt] -> Inverter1/1
  Delay2/1 -> Logical7/2
  Delay/1 -> posedge1/1
  [busy] -> Inverter2/1
  posedge1/1 -> Logical10/2
  [pkt_rdy] -> Delay/1
  [end_of_vector] -> Logical1/2
  Logical10/1 -> Register3/3, Register3/1
  Inverter2/1 -> Logical10/1
  posedge2/1 -> [vector_start]
  Register3/1 -> posedge2/1, [busy]
  Logical8/1 -> Delay3/1
  [pkt_rdy] -> Logical8/1
  Logical4/1 -> Delay4/1
  [vector_start] -> Logical4/1
  [writing_header] -> Inverter/1
  [get_a_pkt] -> Counter4/1
  Convert/1 -> Shift1/1
  AddSub/1 -> Convert/1
  Mult/1 -> AddSub/2
  [xeng_id] -> Mult/1
  Constant5/1 -> Mult/2
  [end_of_vector] -> Delay2/1
  [rb_done] -> Logical7/1
  [err] -> err/1
  [get_a_pkt] -> Register1/2
  Constant1/1 -> Concat1/1
  [heap_cnt] -> Concat1/2
  Register1/1 -> AddSub/1, AddSub1/2
  [vector_position] -> Register1/1
  [writing_header] -> Counter4/2
  Constant4/1 -> Relational3/2
  Relational3/1 -> [writing_header]
  Counter4/1 -> [output_sel], Relational3/1
  [valid_output] -> Logical3/2
  Constant9/1 -> Concat8/1
  [pld_len] -> Concat8/2
  Concat7/1 -> Mux3/6
  Concat1/1 -> Mux3/5
  [heap_offset] -> Concat7/2
  Constant13/1 -> Concat7/1
  Concat6/1 -> Mux3/4
  Constant6/1 -> Concat6/2
  Constant12/1 -> Concat6/1
  Concat5/1 -> Mux3/3
  [heap_cnt] -> Concat5/2
  Constant11/1 -> Concat5/1
  Constant10/1 -> Concat4/1
  Constant22/1 -> Concat4/2
  Concat4/1 -> Mux3/8
  Constant21/1 -> Concat2/6
  Constant20/1 -> Concat2/5
  Delay1/1 -> eof/1
  [eof] -> Delay1/1
  [writing_header] -> Logical3/1
  [data_input] -> Mux3/9
  Constant19/1 -> Concat2/4
  Constant18/1 -> Concat2/3
  Constant17/1 -> Concat2/2
  Constant16/1 -> Concat2/1
  Concat2/1 -> Mux3/2
  [output_sel] -> Mux3/1
  Mux3/1 -> data_out/1, [data_out]
  [vector_position] -> Gateway Out16/1
  [raw_data_input] -> Gateway Out7/1
  [output_sel] -> Gateway Out1/1
  [busy_pkt] -> Gateway Out15/1
  [valid_output] -> Gateway Out8/1
  [busy] -> Gateway Out14/1
  [writing_header] -> Gateway Out9/1
  [fetch_pld] -> Gateway Out6/1
  Relational1/1 -> Logical5/2
  Constant7/1 -> Relational1/2
  [vector_start] -> Counter1/1
  [fetch_pld] -> Counter1/2
  [valid_input] -> Logical6/1
  Logical6/1 -> [valid_output]
  Delay6/1 -> Logical6/2
  Slice3/1 -> Delay6/1
  Gateway Out18/1 -> packetise_output/10
  Gateway Out17/1 -> packetise_output/9
  Delay5/1 -> Concat/1
  rb_done/1 -> Logical2/2
  Reinterpret/1 -> Concat/2, Delay5/1
  pkt_rdy/1 -> [pkt_rdy]
  valid_in/1 -> [valid_input], Logical2/1
  data_in/1 -> [raw_data_input], Reinterpret/1
  Relational5/1 -> [end_of_vector]
  Constant2/1 -> Relational5/2
  [vector_start] -> Register2/2
  Register2/1 -> [heap_cnt]
  timestamp/1 -> Register2/1
  Counter1/1 -> Relational5/1, Slice/1, [vector_position], Slice3/1
  Slice/1 -> Relational1/1
  Gateway Out16/1 -> packetise_output/8
  Concat/1 -> [data_input]
  xeng_id/1 -> [xeng_id]
  Logical2/1 -> [rb_done]
  Logical5/1 -> [eof]
  Gateway Out7/1 -> packetise_output/1
  Gateway Out8/1 -> packetise_output/2
  Gateway Out1/1 -> packetise_output/3
  Gateway Out6/1 -> packetise_output/4
  Gateway Out9/1 -> packetise_output/5
  Gateway Out15/1 -> packetise_output/6
  [end_of_vector] -> Logical5/1
  Gateway Out14/1 -> packetise_output/7

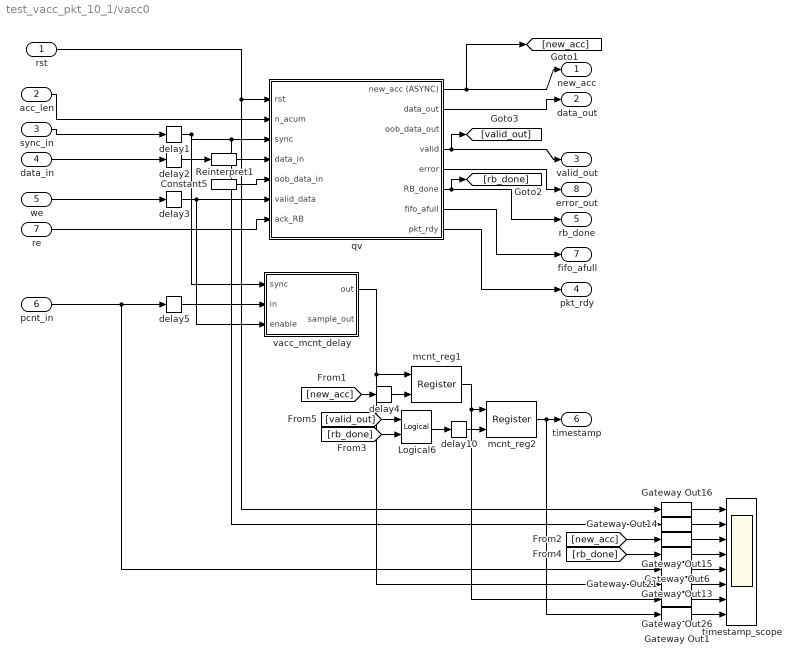
== system test_vacc_pkt_10_1/vacc0 ==
  rst : Inport
  acc_len : Inport  Port=2
  sync_in : Inport  Port=3
  data_in : Inport  Port=4
  we : Inport  Port=5
  pcnt_in : Inport  Port=6
  re : Inport  Port=7
  Constant5 : xbsIndex_r4/Constant  arith_type=Unsigned  const=0  n_bits=4  bin_pt=0  explicit_period=on  period=1  equ=P=C  opselect=C  inp2=PCIN>>17  opr=+  inp1=P  carry=CIN  dbl_ovrd=off  block_type=constant
  Gateway Out{1,6,13..16,21,26} (8 alike) : xbsIndex_r4/Gateway Out  hdl_port=off  timing_constraint=None  locs_specified=off  LOCs={}  block_type=gatewayout
      settings: infoedit="Gateway out block.  Converts Xilinx fixed point inputs into ouputs of type Simulink integer, double, or fixed point.<P><P>Hardware notes:  In hardware these blocks become top level output ports or are discarded, depending on how they are configured."  xl_area=[0, 0, 0, 0, 0, 0, 0]  block_version=10.1.3
  Logical6 : xbsIndex_r4/Logical  logical_function=AND  inputs=2  en=off  latency=0  precision=Full  arith_type=Unsigned  n_bits=16  bin_pt=0  align_bp=on  dbl_ovrd=off  block_type=logical
  Reinterpret1 : xbsIndex_r4/Reinterpret  force_arith_type=on  arith_type="Signed  (2's comp)"  force_bin_pt=on  bin_pt=0  block_type=reinterpret
      settings: infoedit="Changes signal type without altering the binary representation.   You can changed the signal between signed and unsigned, and relocate the binary point.<P><P>Hardware notes: In hardware this block costs nothing.<P><P>Example:  Suppose the input is 6 bits wide, signed, with 2 fractional bits, and the output is forced to unsigned with 0 fractional bits.  Then an input of -2.0 (1110.00 in binary 2's complement) becomes an output of 56 (111000 in binary)."  block_version=10.1.3
  delay{1..3,5} (4 alike) : xbsIndex_r4/Delay  en=off  latency=2  dbl_ovrd=off  reg_retiming=on  block_type=delay
  delay10 : xbsIndex_r4/Delay  en=off  latency=1  dbl_ovrd=off  reg_retiming=on  block_type=delay
  delay4 : xbsIndex_r4/Delay  en=off  latency=1  dbl_ovrd=off  reg_retiming=on  block_type=delay
  mcnt_reg1 : xbsIndex_r4/Register  init=0  rst=off  en=on  dbl_ovrd=off  block_type=register
  mcnt_reg2 : xbsIndex_r4/Register  init=0  rst=off  en=on  dbl_ovrd=off  block_type=register
  qv : Subsystem  mask{vector_len=vector_len, which_qdr=qdr0}
      mask prompts: vector_len "Vector length??(# cycles)"; which_qdr "Which QDR?"
      mask help:
      | A vector accumulator for medium length vectors designed for ROACH's QDR memory.
      |
      | Originally designed for the packetised correlator, this block accepts input data of type Fix_32_0. OOB_data_in provides an extra 4 bits that are accumulated seperately (originally designed to keep track of how many "bad" values in a vector were accumulated).
      |
      | Minimum vector length is 2 * burst_length.
      | Minimum burst length is 10 (recommended default is 2^4=16).
      |
      | The vector length does not need to be a multiple of the burst length.
      mask init:
      | vector_bits = ceil(log2(vector_len));
      | burst_bits = 4;
      | burst_len = 2^burst_bits;
      | set_param([gcb, '/qdr'], 'which_qdr', which_qdr);
      | 
      | fmtstr = sprintf('Vector Length: %d', vector_len);
      | set_param(gcb, 'AttributesFormatString', fmtstr);
      settings: AttributesFormatString=Vector Length: 100
      mask StyleString: edit,popup(qdr0|qdr1)
  timestamp_scope : Scope  NumInputPorts=8
      settings: YMin=0~0~0~0~0~0~0~-5  YMax=800~1~1~1~1~17500~1~5  SaveName=ScopeData13
  vacc_mcnt_delay : Subsystem  mask(sample_and_hold){period=vector_len}
      mask prompts: period "Sample period (clocks)"
      mask help: This block will sample an input signal at a user specified rate and hold the value on the output.
  new_acc : Outport
  data_out : Outport  Port=2
  valid_out : Outport  Port=3
  pkt_rdy : Outport  Port=4
  rb_done : Outport  Port=5
  timestamp : Outport  Port=6
  fifo_afull : Outport  Port=7
  error_out : Outport  Port=8
  wires:
  delay1/1 -> vacc_mcnt_delay/1(sync), qv/3(sync), Gateway Out14/1
  delay5/1 -> vacc_mcnt_delay/2(in)
  delay3/1 -> vacc_mcnt_delay/3(enable), qv/6(valid_data)
  delay2/1 -> Reinterpret1/1
  Reinterpret1/1 -> qv/4(data_in)
  Constant5/1 -> qv/5(oob_data_in)
  qv/1(new_acc (ASYNC)) -> new_acc/1, [new_acc]
  acc_len/1 -> qv/2(n_acum)
  qv/2(data_out) -> data_out/1
  sync_in/1 -> delay1/1
  data_in/1 -> delay2/1
  qv/4(valid) -> valid_out/1, [valid_out]
  qv/5(error) -> error_out/1
  we/1 -> delay3/1
  qv/6(RB_done) -> rb_done/1, [rb_done]
  re/1 -> qv/7(ack_RB)
  qv/7(fifo_afull) -> fifo_afull/1
  pcnt_in/1 -> delay5/1, Gateway Out13/1
  mcnt_reg2/1 -> timestamp/1, Gateway Out1/1
  rst/1 -> qv/1(rst), Gateway Out16/1
  qv/8(pkt_rdy) -> pkt_rdy/1
  [new_acc] -> delay4/1
  delay4/1 -> mcnt_reg1/2
  mcnt_reg1/1 -> mcnt_reg2/1, Gateway Out26/1
  delay10/1 -> mcnt_reg2/2
  vacc_mcnt_delay/1(out) -> mcnt_reg1/1, Gateway Out21/1
  Gateway Out13/1 -> timestamp_scope/5
  Gateway Out6/1 -> timestamp_scope/4
  Gateway Out16/1 -> timestamp_scope/1
  Gateway Out14/1 -> timestamp_scope/2
  Gateway Out15/1 -> timestamp_scope/3
  Gateway Out21/1 -> timestamp_scope/6
  Gateway Out26/1 -> timestamp_scope/7
  [new_acc] -> Gateway Out15/1
  [rb_done] -> Gateway Out6/1
  Gateway Out1/1 -> timestamp_scope/8
  Logical6/1 -> delay10/1
  [rb_done] -> Logical6/2
  [valid_out] -> Logical6/1

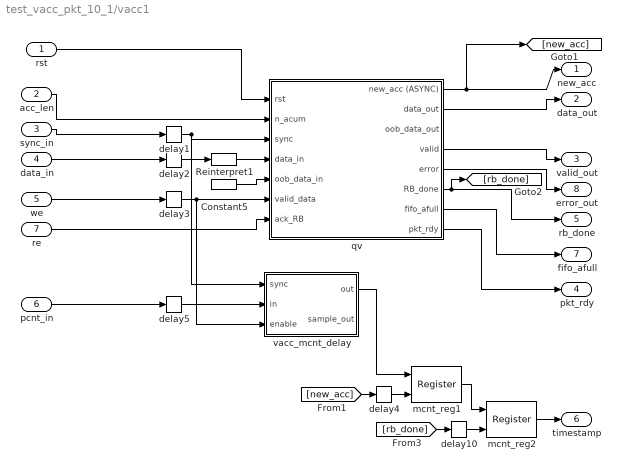
== system test_vacc_pkt_10_1/vacc1 ==
  rst : Inport
  acc_len : Inport  Port=2
  sync_in : Inport  Port=3
  data_in : Inport  Port=4
  we : Inport  Port=5
  pcnt_in : Inport  Port=6
  re : Inport  Port=7
  Constant5 : xbsIndex_r4/Constant  arith_type=Unsigned  const=0  n_bits=4  bin_pt=0  explicit_period=on  period=1  equ=P=C  opselect=C  inp2=PCIN>>17  opr=+  inp1=P  carry=CIN  dbl_ovrd=off  block_type=constant
  Reinterpret1 : xbsIndex_r4/Reinterpret  force_arith_type=on  arith_type="Signed  (2's comp)"  force_bin_pt=on  bin_pt=0  block_type=reinterpret
      settings: infoedit="Changes signal type without altering the binary representation.   You can changed the signal between signed and unsigned, and relocate the binary point.<P><P>Hardware notes: In hardware this block costs nothing.<P><P>Example:  Suppose the input is 6 bits wide, signed, with 2 fractional bits, and the output is forced to unsigned with 0 fractional bits.  Then an input of -2.0 (1110.00 in binary 2's complement) becomes an output of 56 (111000 in binary)."  block_version=10.1.3
  delay{1..3,5} (4 alike) : xbsIndex_r4/Delay  en=off  latency=2  dbl_ovrd=off  reg_retiming=on  block_type=delay
  delay10 : xbsIndex_r4/Delay  en=off  latency=1  dbl_ovrd=off  reg_retiming=on  block_type=delay
  delay4 : xbsIndex_r4/Delay  en=off  latency=1  dbl_ovrd=off  reg_retiming=on  block_type=delay
  mcnt_reg1 : xbsIndex_r4/Register  init=0  rst=off  en=on  dbl_ovrd=off  block_type=register
  mcnt_reg2 : xbsIndex_r4/Register  init=0  rst=off  en=on  dbl_ovrd=off  block_type=register
  qv : Subsystem  mask{vector_len=vector_len, which_qdr=qdr0}
      mask prompts: vector_len "Vector length??(# cycles)"; which_qdr "Which QDR?"
      mask help:
      | A vector accumulator for medium length vectors designed for ROACH's QDR memory.
      |
      | Originally designed for the packetised correlator, this block accepts input data of type Fix_32_0. OOB_data_in provides an extra 4 bits that are accumulated seperately (originally designed to keep track of how many "bad" values in a vector were accumulated).
      |
      | Minimum vector length is 2 * burst_length.
      | Minimum burst length is 10 (recommended default is 2^4=16).
      |
      | The vector length does not need to be a multiple of the burst length.
      mask init: same as test_vacc_pkt_10_1/vacc0/qv
      settings: AttributesFormatString=Vector Length: 100
      mask StyleString: edit,popup(qdr0|qdr1)
  vacc_mcnt_delay : Subsystem  mask(sample_and_hold){period=vector_len}
      mask prompts: period "Sample period (clocks)"
      mask help: This block will sample an input signal at a user specified rate and hold the value on the output.
  new_acc : Outport
  data_out : Outport  Port=2
  valid_out : Outport  Port=3
  pkt_rdy : Outport  Port=4
  rb_done : Outport  Port=5
  timestamp : Outport  Port=6
  fifo_afull : Outport  Port=7
  error_out : Outport  Port=8
  wires:
  vacc_mcnt_delay/1(out) -> mcnt_reg1/1
  delay10/1 -> mcnt_reg2/2
  [rb_done] -> delay10/1
  mcnt_reg1/1 -> mcnt_reg2/1
  delay4/1 -> mcnt_reg1/2
  [new_acc] -> delay4/1
  qv/8(pkt_rdy) -> pkt_rdy/1
  rst/1 -> qv/1(rst)
  mcnt_reg2/1 -> timestamp/1
  pcnt_in/1 -> delay5/1
  qv/7(fifo_afull) -> fifo_afull/1
  re/1 -> qv/7(ack_RB)
  qv/6(RB_done) -> [rb_done], rb_done/1
  we/1 -> delay3/1
  qv/5(error) -> error_out/1
  qv/4(valid) -> valid_out/1
  data_in/1 -> delay2/1
  sync_in/1 -> delay1/1
  qv/2(data_out) -> data_out/1
  acc_len/1 -> qv/2(n_acum)
  qv/1(new_acc (ASYNC)) -> [new_acc], new_acc/1
  Constant5/1 -> qv/5(oob_data_in)
  Reinterpret1/1 -> qv/4(data_in)
  delay2/1 -> Reinterpret1/1
  delay3/1 -> qv/6(valid_data), vacc_mcnt_delay/3(enable)
  delay5/1 -> vacc_mcnt_delay/2(in)
  delay1/1 -> qv/3(sync), vacc_mcnt_delay/1(sync)
